simulink model "Battery_Simulator"  (R2014a)
settings: Solver=FixedStepDiscrete  StartTime=0.0  StopTime=10.0  RelTol=1e-3
PreLoadFcn:
  | try, eval([bdroot '_setup']); catch, eval('model_setup', ''); end
InitFcn:
  | try, eval([bdroot '_setup']); catch, eval('model_setup', ''); end
undefined symbols (not defined in the file or in its folder): ECU565, motohawk_build_version, motohawk_trunc_name, motohawk_vardec_path
undefined symbols (not defined in the file): motohawk_get_target_image, motohawk_target_type
libraries: MotoHawk_lib x42, motohawk_annotations_lib x36
(part 2 of 2)

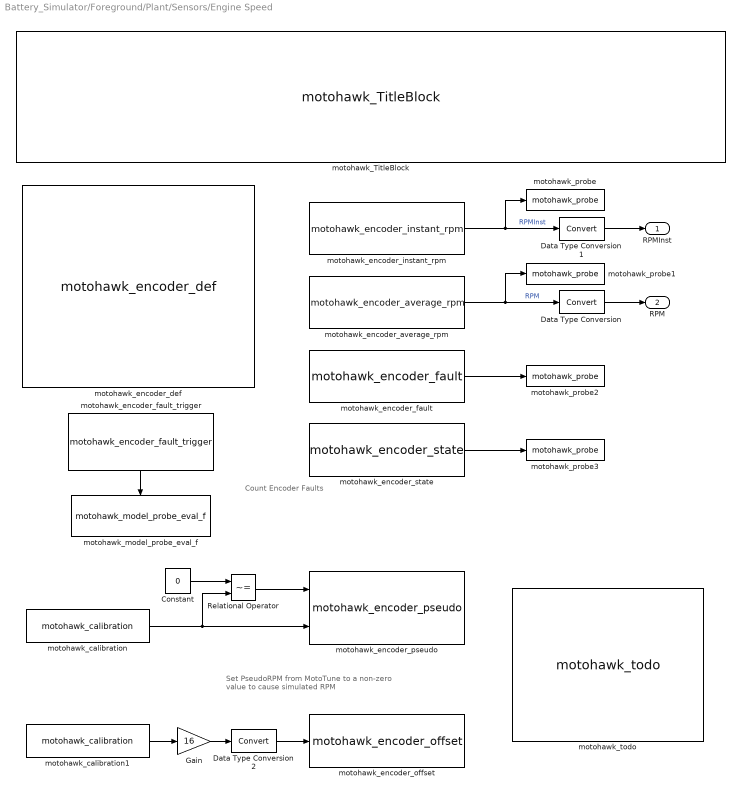
== system Battery_Simulator/Foreground/Plant/Sensors/Engine Speed ==
  note: Set PseudoRPM from MotoTune
      | to a non-zero value to cause
      | simulated RPM
  note: Count
      | Encoder
      | Faults
  Constant : Constant  Value=0  OutDataTypeStr=Inherit: Inherit via back propagation
  Data Type Conversion : DataTypeConversion  SaturateOnIntegerOverflow=on  RndMeth=Zero
  Data Type Conversion1 : DataTypeConversion  SaturateOnIntegerOverflow=on  RndMeth=Zero
  Data Type Conversion2 : DataTypeConversion  SaturateOnIntegerOverflow=on  RndMeth=Zero
  Gain : Gain  Gain=16  OutDataTypeStr=Inherit: Same as input  ParamDataTypeStr=Inherit: Same as input
  Relational Operator : RelationalOperator  Operator=~=  ZeroCross=off  InputSameDT=on
  motohawk_TitleBlock : motohawk_annotations_lib/motohawk_TitleBlock  BlockType_='Mototron_Title_Block'  ttl=[get_param(bdroot, 'Description') '\rm\newlineEngine Encoder Interface\newlineOutput RPM for use in the controller\newline']  copyright="'THE INFORMATION CONTAINED IN THIS\\newlineDRAWING IS THE SOLE PROPERTY OF\\newlineWOODWARD.  ANY REPRODUCTION IN\\newline PART OR AS A WHOLE WITHOUT THE\\newlineWRITTEN PERMISSION OF WOODWARD\\newline IS PROHIBITED.\\fontsize{16}\\rm\\copyright\\rm\\fontsize{10} 2009'"  address='\fontsize{22}\it\fontname{Arial Black}Woodward \fontname{Arial}\fontsize{10}\newline1000 East Drake Road, Fort Collins, CO, 80525\newlinemcs.woodward.com (866) 588-0494'  image_file='mh.jpg'  pretty_print=on  edit_text=|  edit_as=6
      | [get_param(bdroot, 'Description') '\rm
      | 
      | 
      | Engine Encoder Interface
      | 
      | 
      | Output RPM for use in the controller
      | 
      | 
      | ']
  motohawk_calibration : MotoHawk_lib/Calibration & Probing Blocks/motohawk_calibration  nam='PseudoRPM'  val=0  storage=Display  show_more=on  name_source=Use Parameter  data_type=Inherit via back propagation  read_level=1  write_level=1  ovr_cals=on  view_as=Number  enum_struct={'Disabled', 'Enabled'}  vector_style=Wide Row  use_help_units=off  help=''  units=''  use_header_enum=off  row_header_enum={}  col_header_enum={}  use_min_max=off  min_val=-inf  max_val=inf  use_precision=off  precision=''  gain=1  offset=0  exp=1  use_mototune_group=off  mototune_group=motohawk_vardec_path(gcb)  data_stores=motohawk_sfun_calibration_data_stores
  motohawk_calibration1 : MotoHawk_lib/Calibration & Probing Blocks/motohawk_calibration  nam='EncoderTDCOffset'  val=0  storage=Calibration  show_more=on  name_source=Use Parameter  data_type=Inherit via back propagation  read_level=1  write_level=1  ovr_cals=on  view_as=Number  enum_struct={'Disabled', 'Enabled'}  vector_style=Wide Row  use_help_units=on  help="'TDC offset of crank sensor, in degrees before TDC1.  Used to align sensor with crank angle.'"  units='degCA'  use_header_enum=off  row_header_enum={}  col_header_enum={}  use_min_max=on  min_val=0  max_val=720  use_precision=off  precision=''  gain=1  offset=0  exp=1  use_mototune_group=on  mototune_group='System | Encoder | Encoder Config'  data_stores=motohawk_sfun_calibration_data_stores
  motohawk_encoder_average_rpm : MotoHawk_lib/Encoder Blocks/motohawk_encoder_average_rpm  resolution=1
  motohawk_encoder_def : MotoHawk_lib/Encoder Blocks/motohawk_encoder_def  encoder_type=60 Minus 2 - 4-Stroke - No CAM  interface=VR Crank  sync=Falling Edge  crnkpullup=Weak Pullup  camsync=Rising Edge  campullup=Weak Pullup  angle_offset=0  sec_tdcoffset=-34.3  cam_delay=0  teeth_after_cam=-1  ignore_teeth=0  ignore_delay=0  angles=[0 360 180 540]  cnk_align_with_cam=off  adaptive_vr_cnk=off  adaptive_vr_cam=on  cal_cylinders=on  max_cylinders=8  num_cylinders=4  read_level=1  write_level=1  ovr_cals=on  group='System | Encoder'
  motohawk_encoder_fault : MotoHawk_lib/Encoder Blocks/motohawk_encoder_fault
  motohawk_encoder_fault_trigger : MotoHawk_lib/Encoder Blocks/motohawk_encoder_fault_trigger  Tag=Trigger  trig_name=[]  inherited=off
  motohawk_encoder_instant_rpm : MotoHawk_lib/Encoder Blocks/motohawk_encoder_instant_rpm  resolution=1
  motohawk_encoder_offset : MotoHawk_lib/Encoder Blocks/motohawk_encoder_offset
  motohawk_encoder_pseudo : MotoHawk_lib/Encoder Blocks/motohawk_encoder_pseudo
  motohawk_encoder_state : MotoHawk_lib/Encoder Blocks/motohawk_encoder_state
  motohawk_model_probe_eval_f : MotoHawk_lib/Extra Development Blocks/motohawk_model_probe_eval_f  nam='EncoderFaultCount'  group=motohawk_vardec_path(gcb)
  motohawk_probe : MotoHawk_lib/Calibration & Probing Blocks/motohawk_probe  nam='RPMInst'  show_more=on  name_source=Use Input Wire Name  read_level=1  view_as=Number  enum_struct={'Disabled', 'Enabled'}  vector_style=Wide Row  use_help_units=off  help=''  units=''  use_header_enum=off  row_header_enum={}  col_header_enum={}  use_min_max=off  min_val=-inf  max_val=inf  use_precision=off  precision=''  gain=1  offset=0  exp=1  use_mototune_group=off  mototune_group=motohawk_vardec_path(gcb)
  motohawk_probe1 : MotoHawk_lib/Calibration & Probing Blocks/motohawk_probe  nam='RPM'  show_more=on  name_source=Use Input Wire Name  read_level=1  view_as=Number  enum_struct={'Disabled', 'Enabled'}  vector_style=Wide Row  use_help_units=off  help=''  units=''  use_header_enum=off  row_header_enum={}  col_header_enum={}  use_min_max=off  min_val=-inf  max_val=inf  use_precision=off  precision=''  gain=1  offset=0  exp=1  use_mototune_group=off  mototune_group=motohawk_vardec_path(gcb)
  motohawk_probe2 : MotoHawk_lib/Calibration & Probing Blocks/motohawk_probe  nam='EncoderFault'  show_more=on  name_source=Use Parameter  read_level=1  view_as=Enumeration  enum_struct={'OK', 'Crank Sync Fault', 'Reverse Rotation', 'No Crank Edges', 'No CAM Edges', 'CAM Sync Fault','Encoder Sync Error on Slave','Reverse Rotation on Slave','Slave Encoder Loss'}  vector_style=Wide Row  use_help_units=on  help='Encoder synchronization fault status'  units=''  use_header_enum=off  row_header_enum={}  col_header_enum={}  use_min_max=off  min_val=-inf  max_val=inf  use_precision=off  precision=''  gain=1  offset=0  exp=1  use_mototune_group=off  mototune_group=motohawk_vardec_path(gcb)
  motohawk_probe3 : MotoHawk_lib/Calibration & Probing Blocks/motohawk_probe  nam='EncoderState'  show_more=on  name_source=Use Parameter  read_level=1  view_as=Enumeration  enum_struct={'', 'Zero Speed', 'Position Unknown', 'Crank Sync - CAM Unknown', 'Crank Sync - CAM Sync', 'Crank Sync - Master Only', 'Crank Sync - Slave Only', 'Crank Sync - Master + Slave'}  vector_style=Wide Row  use_help_units=on  help='Encoder synchronization status'  units=''  use_header_enum=off  row_header_enum={}  col_header_enum={}  use_min_max=off  min_val=-inf  max_val=inf  use_precision=off  precision=''  gain=1  offset=0  exp=1  use_mototune_group=off  mototune_group=motohawk_vardec_path(gcb)
  motohawk_todo : motohawk_annotations_lib/motohawk_todo  BlockType_='Mototron_ToDo'  desc='\fontsize{16}\bfTo Do:\newlineSetup encoder interface\newlinefor a specific engine'  edit_text=|  edit_as=2
      | \fontsize{16}\bfTo Do:
      | 
      | 
      | Setup encoder interface
      | 
      | 
      | for a specific engine
  RPMInst : Outport
  RPM : Outport  Port=2
  wires:
  motohawk_encoder_instant_rpm/1 -> motohawk_probe/1, Data Type Conversion1/1  "RPMInst"
  motohawk_encoder_average_rpm/1 -> motohawk_probe1/1, Data Type Conversion/1  "RPM"
  motohawk_calibration/1 -> motohawk_encoder_pseudo/2, Relational Operator/2
  Relational Operator/1 -> motohawk_encoder_pseudo/1
  Constant/1 -> Relational Operator/1
  Data Type Conversion/1 -> RPM/1
  Data Type Conversion1/1 -> RPMInst/1
  motohawk_encoder_fault/1 -> motohawk_probe2/1
  motohawk_calibration1/1 -> Gain/1
  Gain/1 -> Data Type Conversion2/1
  Data Type Conversion2/1 -> motohawk_encoder_offset/1
  motohawk_encoder_state/1 -> motohawk_probe3/1
  motohawk_encoder_fault_trigger/1 -> motohawk_model_probe_eval_f/Trigger

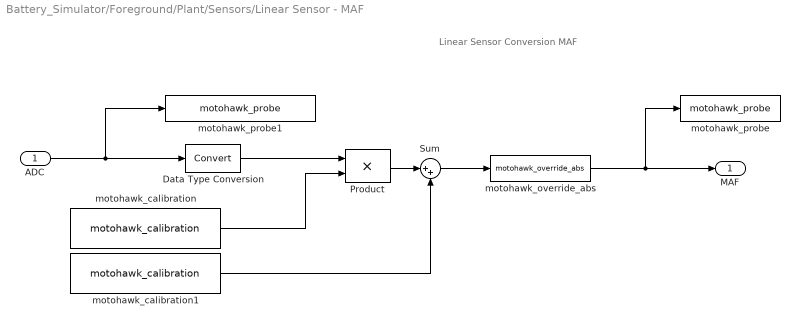
== system Battery_Simulator/Foreground/Plant/Sensors/Linear Sensor - MAF ==
  note: Linear Sensor Conversion
      | MAF
  ADC : Inport
  Data Type Conversion : DataTypeConversion  SaturateOnIntegerOverflow=on  RndMeth=Zero
  Product : Product  InputSameDT=on  OutDataTypeStr=Inherit: Same as first input
  Sum : Sum  Inputs=|++  InputSameDT=on
  motohawk_calibration : MotoHawk_lib/Calibration & Probing Blocks/motohawk_calibration  nam='MAF_Gain'  val=1  storage=Calibration  show_more=off  name_source=Use Parameter  data_type=Inherit from 'Default Value'  read_level=1  write_level=1  ovr_cals=on  view_as=Number  enum_struct={'Disabled', 'Enabled'}  vector_style=Wide Row  use_help_units=off  help=''  units=''  use_header_enum=off  row_header_enum={}  col_header_enum={}  use_min_max=off  min_val=-inf  max_val=inf  use_precision=off  precision=''  gain=1  offset=0  exp=1  use_mototune_group=off  mototune_group=motohawk_vardec_path(gcb)  data_stores=motohawk_sfun_calibration_data_stores
  motohawk_calibration1 : MotoHawk_lib/Calibration & Probing Blocks/motohawk_calibration  nam='MAF_Offset'  val=0  storage=Calibration  show_more=off  name_source=Use Parameter  data_type=Inherit from 'Default Value'  read_level=1  write_level=1  ovr_cals=on  view_as=Number  enum_struct={'Disabled', 'Enabled'}  vector_style=Wide Row  use_help_units=off  help=''  units=''  use_header_enum=off  row_header_enum={}  col_header_enum={}  use_min_max=off  min_val=-inf  max_val=inf  use_precision=off  precision=''  gain=1  offset=0  exp=1  use_mototune_group=off  mototune_group=motohawk_vardec_path(gcb)  data_stores=motohawk_sfun_calibration_data_stores
  motohawk_override_abs : MotoHawk_lib/Calibration & Probing Blocks/motohawk_override_abs  parent_name='MAF'  parent_val=0  show_more=off  name_source=Use Parameter  parent_read_level=1  parent_override_level=1  view_as=Number  enum_struct={'Disabled', 'Enabled'}  use_help_units=off  parent_help=''  parent_units=''  use_min_max=off  parent_min=-inf  parent_max=inf  use_precision=off  parent_precision=''  parent_gain=1  parent_offset=0  parent_exp=1  use_mototune_group=off  parent_group=motohawk_vardec_path(gcb)
  motohawk_probe : MotoHawk_lib/Calibration & Probing Blocks/motohawk_probe  nam='MAF'  show_more=off  name_source=Use Parameter  read_level=1  view_as=Number  enum_struct={'Disabled', 'Enabled'}  vector_style=Wide Row  use_help_units=off  help=''  units=''  use_header_enum=off  row_header_enum={}  col_header_enum={}  use_min_max=off  min_val=-inf  max_val=inf  use_precision=off  precision=''  gain=1  offset=0  exp=1  use_mototune_group=off  mototune_group=motohawk_vardec_path(gcb)
  motohawk_probe1 : MotoHawk_lib/Calibration & Probing Blocks/motohawk_probe  nam='MAF_ADC'  show_more=off  name_source=Use Parameter  read_level=1  view_as=Number  enum_struct={'Disabled', 'Enabled'}  vector_style=Wide Row  use_help_units=off  help=''  units=''  use_header_enum=off  row_header_enum={}  col_header_enum={}  use_min_max=off  min_val=-inf  max_val=inf  use_precision=off  precision=''  gain=1  offset=0  exp=1  use_mototune_group=off  mototune_group=motohawk_vardec_path(gcb)
  MAF : Outport
  wires:
  motohawk_calibration/1 -> Product/2
  Product/1 -> Sum/1
  motohawk_calibration1/1 -> Sum/2
  Data Type Conversion/1 -> Product/1
  ADC/1 -> Data Type Conversion/1, motohawk_probe1/1
  Sum/1 -> motohawk_override_abs/1
  motohawk_override_abs/1 -> MAF/1, motohawk_probe/1

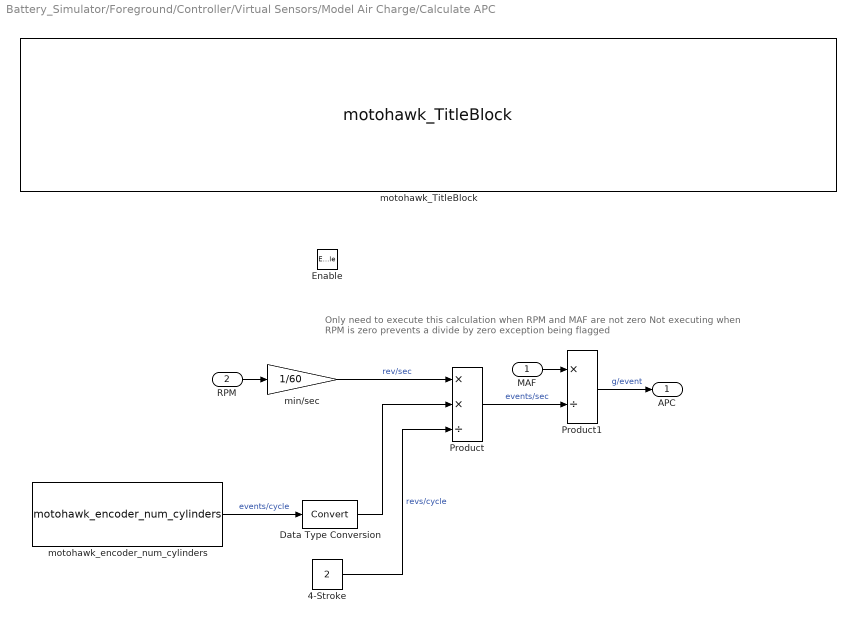
== system Battery_Simulator/Foreground/Controller/Virtual Sensors/Model Air Charge/Calculate APC ==
  note: Only need to execute this calculation when RPM and MAF are not zero
      | Not executing when RPM is zero prevents a divide by zero exception being flagged
  MAF : Inport
  RPM : Inport  Port=2
  Enable : EnablePort
  4-Stroke : Constant  Value=2
  Data Type Conversion : DataTypeConversion  SaturateOnIntegerOverflow=on  RndMeth=Zero
  Product : Product  Inputs=**/  InputSameDT=on  OutDataTypeStr=Inherit: Same as first input
  Product1 : Product  Inputs=*/  SaturateOnIntegerOverflow=on  OutDataTypeStr=Inherit: Same as first input
  min/sec : Gain  Gain=1/60  OutDataTypeStr=Inherit: Same as input  ParamDataTypeStr=Inherit: Same as input
  motohawk_TitleBlock : motohawk_annotations_lib/motohawk_TitleBlock  BlockType_='Mototron_Title_Block'  ttl=[get_param(bdroot, 'Description') '\rm\newlineCompute Air Charge per Cylinder\newline(Grams / Event)\newline']  copyright="'THE INFORMATION CONTAINED IN THIS\\newlineDRAWING IS THE SOLE PROPERTY OF\\newlineWOODWARD.  ANY REPRODUCTION IN\\newline PART OR AS A WHOLE WITHOUT THE\\newlineWRITTEN PERMISSION OF WO0DWARD\\newline IS PROHIBITED.\\fontsize{16}\\rm\\copyright\\rm\\fontsize{10} 2009'"  address='\fontsize{22}\it\fontname{Arial Black}Woodward \fontname{Arial}\fontsize{10}\newline1000 East Drake Road, Fort Collins, CO, 80525\newlinemcs.woodward.com (866) 588-0494'  image_file='mh.jpg'  pretty_print=on  edit_text=|  edit_as=6
      | [get_param(bdroot, 'Description') '\rm
      | 
      | 
      | Compute Air Charge per Cylinder
      | 
      | 
      | (Grams / Event)
      | 
      | 
      | ']
  motohawk_encoder_num_cylinders : MotoHawk_lib/Encoder Blocks/motohawk_encoder_num_cylinders
  APC : Outport
  wires:
  motohawk_encoder_num_cylinders/1 -> Data Type Conversion/1  "events/cycle"
  min/sec/1 -> Product/1  "rev/sec"
  Product/1 -> Product1/2  "events/sec"
  4-Stroke/1 -> Product/3  "revs/cycle"
  Data Type Conversion/1 -> Product/2
  MAF/1 -> Product1/1
  Product1/1 -> APC/1  "g/event"
  RPM/1 -> min/sec/1
